simulink model "B64SNSTest"  (R2022a)
settings: Solver=VariableStepAuto  StartTime=0.0  StopTime=40  RelTol=1E-4  AbsTol=1E-4
values from neighbouring files (symbols this model uses):
  AinfKpp_h_B64 = -50    [CtrlParaSNSTuning.m]
  AinfKpp_p_B64 = 1.0    (= 1)    [CtrlParaSNSTuning.m]
  AinfKpp_s_B64 = 1.0    (= 1)    [CtrlParaSNSTuning.m]
  AinfNapp_h_B64 = -50    [CtrlParaSNSTuning.m]
  AinfNapp_p_B64 = 1.0    (= 1)    [CtrlParaSNSTuning.m]
  AinfNapp_s_B64 = 1.0    (= 1)    [CtrlParaSNSTuning.m]
  AKpp_B64_0 = 0.5    [CtrlParaSNSTuning.m]    (also in InitPara.m)
  ANapp_B64_0 = 0.5    [CtrlParaSNSTuning.m]    (also in InitPara.m)
  Cm_B64 = 0.01    [CtrlParaSNSTuning.m]
  EKpp_B64 = -70    [CtrlParaSNSTuning.m]
  EL_B64 = -60    [CtrlParaSNSTuning.m]
  ENapp_B64 = 30    [CtrlParaSNSTuning.m]
  gKpp_B64 = 0.35    [CtrlParaSNSTuning.m]
  gL_B64 = 0.1927    [CtrlParaSNSTuning.m]    (also in ModularAplysia_1282022_withSNS_initialization.m)
  gNapp_B64 = 0.1    [CtrlParaSNSTuning.m]
  pKpp_B64 = 1    [CtrlParaSNSTuning.m]
  pNapp_B64 = 1    [CtrlParaSNSTuning.m]
  sigmarinf = 2.5    [B34.m]    (also in CtrlParaSNSTuning.m)
  tAKpp_t_B64 = 4    [CtrlParaSNSTuning.m]
  tANapp_t_B64 = 0.1    [CtrlParaSNSTuning.m]
  thetarinf = 40    [B34.m]    (also in CtrlParaSNSTuning.m = 43.5)
  V_B64_0 = -60    [CtrlParaSNSTuning.m]    (also in InitPara.m)
undefined symbols (not defined in the file or in its folder): Iapp
settings Model: SimulationMode=accelerator  Creator=liyan  LastModifiedBy=liyan

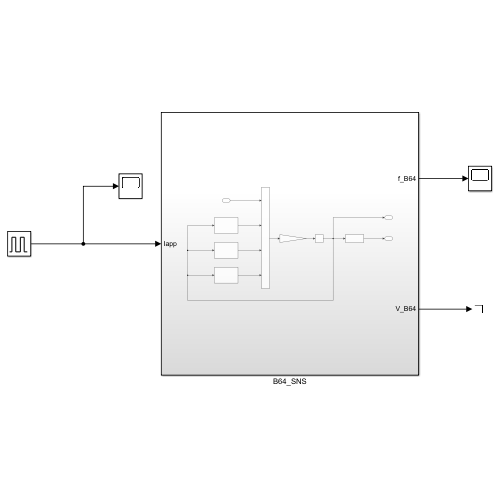
[thumbnail: Simulink's stored preview of the top-level diagram]
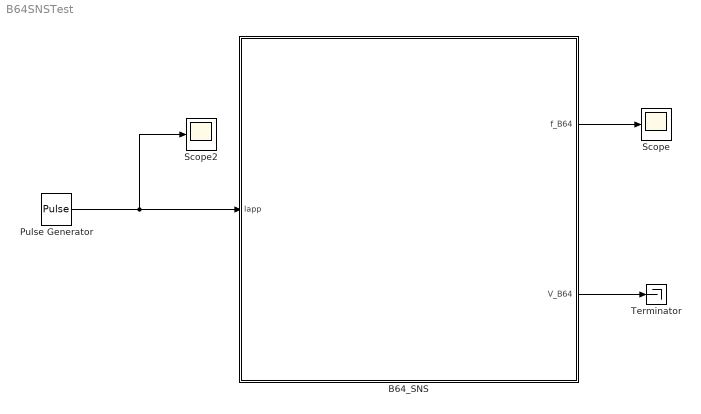
== system B64SNSTest ==
  B64_SNS : Subsystem
  Pulse Generator : DiscretePulseGenerator  PulseType=Time based  Amplitude=Iapp  Period=40  PulseWidth=0.3/40*100  PhaseDelay=30
  Scope : Scope
  Scope2 : Scope
  Terminator : Terminator
  wires:
  Pulse Generator/1 -> Scope2/1, B64_SNS/1(Iapp)
  B64_SNS/1(f_B64) -> Scope/1
  B64_SNS/2(V_B64) -> Terminator/1

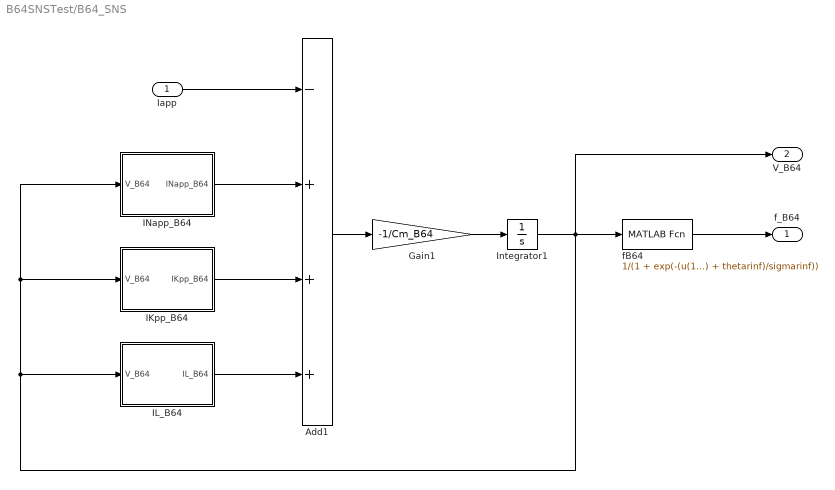
== system B64SNSTest/B64_SNS ==
  Iapp : Inport
  Add1 : Sum  Inputs=-+++
  Gain1 : Gain  Gain=-1/Cm_B64
  IKpp_B64 : Subsystem
  IL_B64 : Subsystem
  INapp_B64 : Subsystem
  Integrator1 : Integrator  InitialCondition=V_B64_0
  fB64 : MATLABFcn  MATLABFcn=1/(1 + exp(-(u(1) + thetarinf)/sigmarinf))
  f_B64 : Outport
  V_B64 : Outport  Port=2
  wires:
  IKpp_B64/1(IKpp_B64) -> Add1/3
  Gain1/1 -> Integrator1/1
  Add1/1 -> Gain1/1
  IL_B64/1(IL_B64) -> Add1/4
  INapp_B64/1(INapp_B64) -> Add1/2
  fB64/1 -> f_B64/1
  Integrator1/1 -> V_B64/1, fB64/1, INapp_B64/1(V_B64), IKpp_B64/1(V_B64), IL_B64/1(V_B64)
  Iapp/1 -> Add1/1

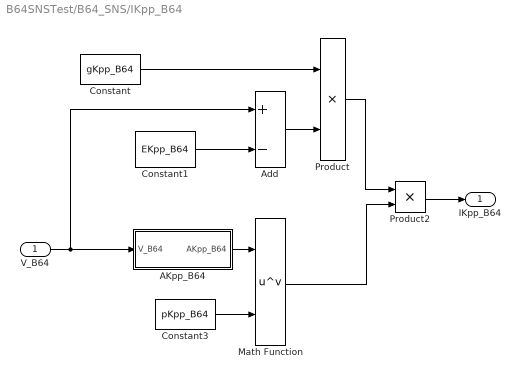
== system B64SNSTest/B64_SNS/IKpp_B64 ==
  V_B64 : Inport
  AKpp_B64 : Subsystem
  Add : Sum  Inputs=+-
  Constant : Constant  Value=gKpp_B64
  Constant1 : Constant  Value=EKpp_B64
  Constant3 : Constant  Value=pKpp_B64
  Math Function : Math  Operator=pow
  Product : Product
  Product2 : Product
  IKpp_B64 : Outport
  wires:
  Add/1 -> Product/2
  Constant1/1 -> Add/2
  V_B64/1 -> AKpp_B64/1(V_B64), Add/1
  Product/1 -> Product2/1
  Math Function/1 -> Product2/2
  Product2/1 -> IKpp_B64/1
  Constant/1 -> Product/1
  AKpp_B64/1(AKpp_B64) -> Math Function/1
  Constant3/1 -> Math Function/2

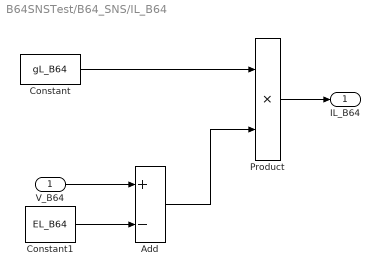
== system B64SNSTest/B64_SNS/IL_B64 ==
  V_B64 : Inport
  Add : Sum  Inputs=+-
  Constant : Constant  Value=gL_B64
  Constant1 : Constant  Value=EL_B64
  Product : Product
  IL_B64 : Outport
  wires:
  Constant1/1 -> Add/2
  V_B64/1 -> Add/1
  Constant/1 -> Product/1
  Add/1 -> Product/2
  Product/1 -> IL_B64/1

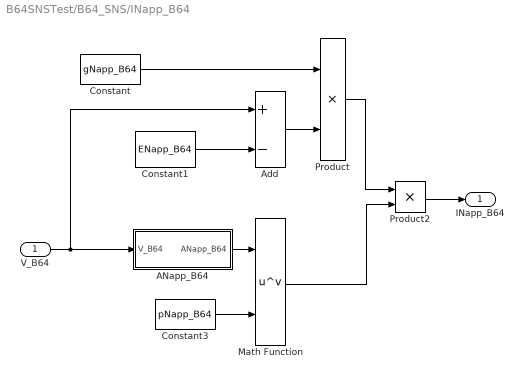
== system B64SNSTest/B64_SNS/INapp_B64 ==
  V_B64 : Inport
  ANapp_B64 : Subsystem
  Add : Sum  Inputs=+-
  Constant : Constant  Value=gNapp_B64
  Constant1 : Constant  Value=ENapp_B64
  Constant3 : Constant  Value=pNapp_B64
  Math Function : Math  Operator=pow
  Product : Product
  Product2 : Product
  INapp_B64 : Outport
  wires:
  Add/1 -> Product/2
  Constant1/1 -> Add/2
  V_B64/1 -> ANapp_B64/1(V_B64), Add/1
  Product/1 -> Product2/1
  Math Function/1 -> Product2/2
  Product2/1 -> INapp_B64/1
  Constant/1 -> Product/1
  ANapp_B64/1(ANapp_B64) -> Math Function/1
  Constant3/1 -> Math Function/2

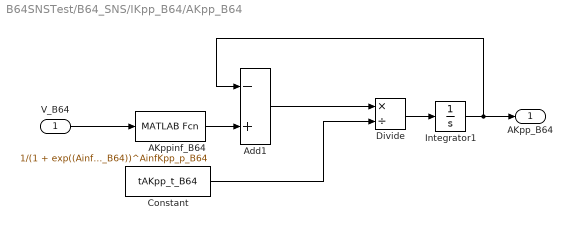
== system B64SNSTest/B64_SNS/IKpp_B64/AKpp_B64 ==
  V_B64 : Inport
  AKppinf_B64 : MATLABFcn  MATLABFcn=1/(1 + exp((AinfKpp_h_B64 - u(1))/AinfKpp_s_B64))^AinfKpp_p_B64
  Add1 : Sum  Inputs=-+
  Constant : Constant  Value=tAKpp_t_B64
  Divide : Product  Inputs=*/
  Integrator1 : Integrator  InitialCondition=AKpp_B64_0
  AKpp_B64 : Outport
  wires:
  Constant/1 -> Divide/2
  Divide/1 -> Integrator1/1
  V_B64/1 -> AKppinf_B64/1
  Integrator1/1 -> Add1/1, AKpp_B64/1
  Add1/1 -> Divide/1
  AKppinf_B64/1 -> Add1/2

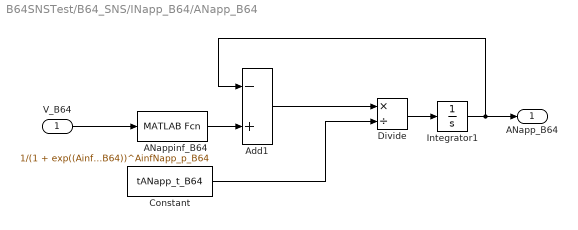
== system B64SNSTest/B64_SNS/INapp_B64/ANapp_B64 ==
  V_B64 : Inport
  ANappinf_B64 : MATLABFcn  MATLABFcn=1/(1 + exp((AinfNapp_h_B64 - u(1))/AinfNapp_s_B64))^AinfNapp_p_B64
  Add1 : Sum  Inputs=-+
  Constant : Constant  Value=tANapp_t_B64
  Divide : Product  Inputs=*/
  Integrator1 : Integrator  InitialCondition=ANapp_B64_0
  ANapp_B64 : Outport
  wires:
  Constant/1 -> Divide/2
  Divide/1 -> Integrator1/1
  V_B64/1 -> ANappinf_B64/1
  Integrator1/1 -> Add1/1, ANapp_B64/1
  Add1/1 -> Divide/1
  ANappinf_B64/1 -> Add1/2
